simulink model "ESTmodel"  (R2025a)
settings: Solver=VariableStepAuto  StartTime=0.0  StopTime=31536000  MaxStep=10  RelTol=1e-6  AbsTol=1e-8
InitFcn:
  | ParametersModel
values from neighbouring files (symbols this model uses):
  P_atm = 101325    [ParametersModel.m]
  P_max = 10000000    [ParametersModel.m]
  P_tank = 132516    [ParametersModel.m]
  R_air = 287    [ParametersModel.m]
  Temp = 293.15    [ParametersModel.m]
  V = 5    [ParametersModel.m]
settings Model: Creator=20253565  LastModifiedBy=20253565

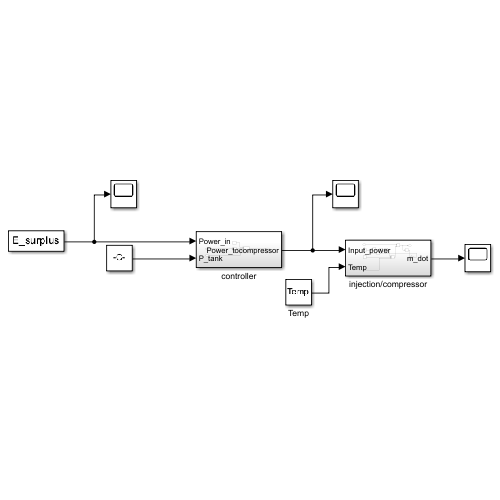
[thumbnail: Simulink's stored preview of the top-level diagram]
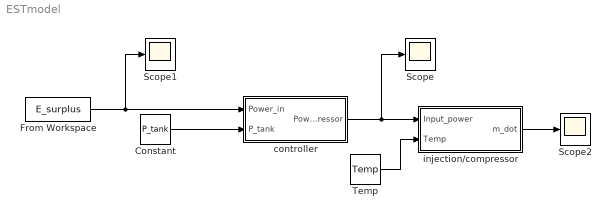
== system ESTmodel ==
  Constant : Constant  Value=P_tank
  From Workspace : FromWorkspace  VariableName=E_surplus  OutputAfterFinalValue=Setting to zero
  Scope : Scope
      settings: ActiveDisplayYMinimum=-2.0826775150843825E+7  ActiveDisplayYMaximum=1.8744097635759446E+8
  Scope1 : Scope
      settings: ActiveDisplayYMinimum=-3.8045691369696744E+7  ActiveDisplayYMaximum=1.3912675683481228E+8
  Scope2 : Scope
      settings: ActiveDisplayYMinimum=-1  ActiveDisplayYMaximum=1  DataLoggingVariableName=ScopeData2
  Temp : Constant  Value=Temp
  controller : Subsystem
  injection/compressor : Subsystem
  wires:
  Temp/1 -> injection/compressor/2(Temp)
  From Workspace/1 -> controller/1(Power_in), Scope1/1
  controller/1(Power_tocompressor) -> Scope/1, injection/compressor/1(Input_power)
  Constant/1 -> controller/2(P_tank)
  injection/compressor/1(m_dot) -> Scope2/1

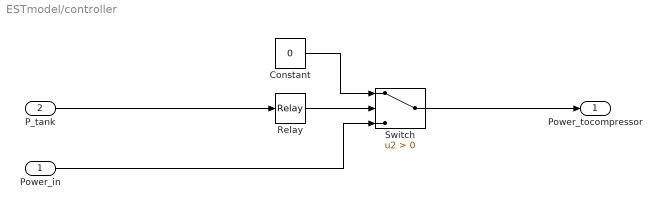
== system ESTmodel/controller ==
  Power_in : Inport
  P_tank : Inport  Port=2
  Constant : Constant  Value=0
  Relay : Relay  OnSwitchValue=P_max  OffSwitchValue=P_max * 0.9
  Switch : Switch  Criteria=u2 > Threshold  SaturateOnIntegerOverflow=off  InputSameDT=off
  Power_tocompressor : Outport
  wires:
  P_tank/1 -> Relay/1
  Relay/1 -> Switch/2
  Constant/1 -> Switch/1
  Power_in/1 -> Switch/3
  Switch/1 -> Power_tocompressor/1

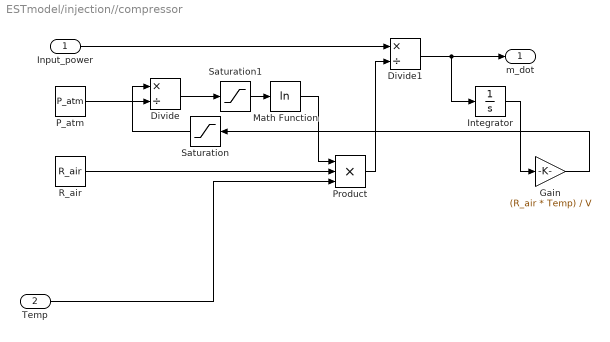
== system ESTmodel/injection//compressor ==
  Input_power : Inport
  Temp : Inport  Port=2
  Divide : Product  Inputs=*/
  Divide1 : Product  Inputs=*/
  Gain : Gain  Gain=(R_air * Temp) / V
  Integrator : Integrator  InitialCondition=1.0
  Math Function : Math  Operator=log
  P_atm : Constant  Value=P_atm
  Product : Product  Inputs=3
  R_air : Constant  Value=R_air
  Saturation : Saturate  LowerLimit=1e-6
  Saturation1 : Saturate  LowerLimit=1e-6
  m_dot : Outport
  wires:
  P_atm/1 -> Divide/2
  Divide/1 -> Saturation1/1
  Math Function/1 -> Product/1
  R_air/1 -> Product/2
  Temp/1 -> Product/3
  Input_power/1 -> Divide1/1
  Product/1 -> Divide1/2
  Divide1/1 -> Integrator/1, m_dot/1
  Integrator/1 -> Gain/1
  Gain/1 -> Saturation/1
  Saturation/1 -> Divide/1
  Saturation1/1 -> Math Function/1
